simulink subsystem "ElectricalThermalSystemSSC"  (R2025b)
settings: Solver=VariableStepAuto  StartTime=0.0  StopTime=10.0  RelTol=1e-3
undefined symbols (not defined in the file): coolant_pipe_D, coolant_valve_D_ratio_max, coolant_valve_D_ratio_min, coolant_valve_displacement, EnvAirTemp, EnvGrvty, PlantThrEstCmpPwr, PlntThrChArea, PlntThrFanMaxSpd, PlntThrFanMechEff, PlntThrFanVolEff, PlntThrHeaterMaxPwr, PlntThrPipeArea, PlntThrPipeDia, PlntThrPmpMaxSpd, PlntThrRadRamEff, PlntThrRefrigAinit, PlntThrTankArea, PlntThrTankVol, PlntThrValDisp, PlntThrValDratioMax, PlntThrValDratioMin, PlntThrValSplMax, ThrmEM1, ThrmEM2, ThrmEM3, ThrmEM4
libraries: fl_lib x159, nesl_utility x69, SimscapeFluids_lib x25, autolibutils x12
(part 5 of 5)

== system ElectricalThermalSystemSSC/Refrigeration Loop/System Level/LPF with IC1 ==
  u : Inport
  Cont LPF IC : autolibutils/Cont LPF IC  wc=wc  aMode=1  dataType=off
  Initial Condition : Constant  Value=InitCond  SampleTime=-1
  y : Outport
  wires:
  Cont LPF IC/1 -> y/1
  u/1 -> Cont LPF IC/1
  Initial Condition/1 -> Cont LPF IC/2

== system ElectricalThermalSystemSSC/Refrigeration Loop/Power Estimate/Environment/LPF with IC1 ==
  u : Inport
  Cont LPF IC : autolibutils/Cont LPF IC  wc=wc  aMode=1  dataType=off
  Initial Condition : Constant  Value=InitCond  SampleTime=-1
  y : Outport
  wires:
  Cont LPF IC/1 -> y/1
  u/1 -> Cont LPF IC/1
  Initial Condition/1 -> Cont LPF IC/2

== system ElectricalThermalSystemSSC/Refrigeration Loop/System Level/Environment/LPF with IC1 ==
  u : Inport
  Cont LPF IC : autolibutils/Cont LPF IC  wc=wc  aMode=1  dataType=off
  Initial Condition : Constant  Value=InitCond  SampleTime=-1
  y : Outport
  wires:
  Cont LPF IC/1 -> y/1
  u/1 -> Cont LPF IC/1
  Initial Condition/1 -> Cont LPF IC/2
